simulink model "fft_1"  (R2019a)
settings: Solver=VariableStepAuto  StartTime=0.0  StopTime=Tsim  RelTol=1e-3
values from neighbouring files (symbols this model uses):
  Fsin = 25    [Script.m]
  Te = T/M    (= 0.03125)    [Script.m]
settings Model: Creator=fleon  LastModifiedBy=fleon

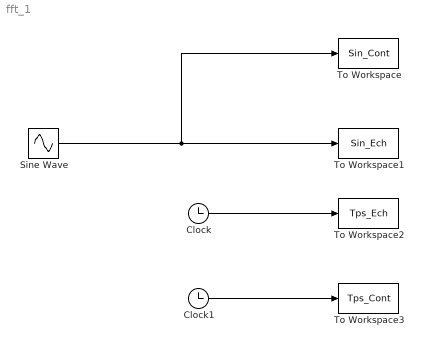
== system fft_1 ==
  Clock : Clock
  Clock1 : Clock
  Sine Wave : Sin  Frequency=2*pi*Fsin  SampleTime=0
  To Workspace : ToWorkspace  VariableName=Sin_Cont  SampleTime=Te/100
  To Workspace1 : ToWorkspace  VariableName=Sin_Ech  SampleTime=Te
  To Workspace2 : ToWorkspace  VariableName=Tps_Ech  SampleTime=Te
  To Workspace3 : ToWorkspace  VariableName=Tps_Cont  SampleTime=Te/100
  wires:
  Sine Wave/1 -> To Workspace/1, To Workspace1/1
  Clock/1 -> To Workspace2/1
  Clock1/1 -> To Workspace3/1
